simulink model "lab2_examples"  (R2022b)
settings: Solver=VariableStepAuto  StartTime=0.0  StopTime=10.0  RelTol=1e-3
settings Model: Creator=gaura  LastModifiedBy=gaura

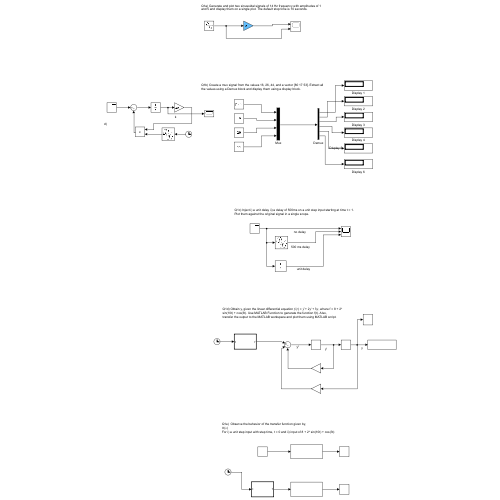
[thumbnail: Simulink's stored preview of the top-level diagram]
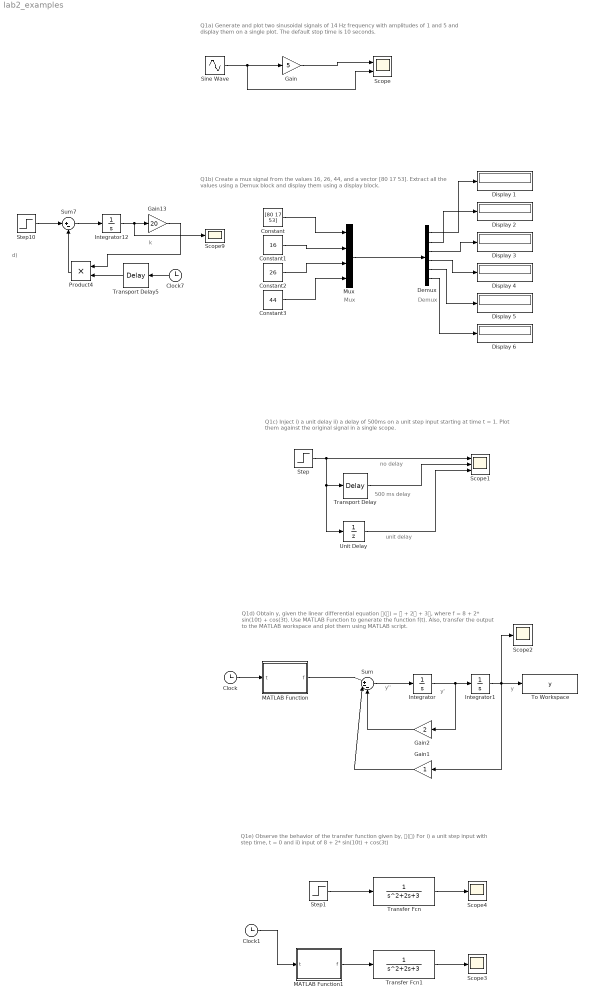
== system lab2_examples ==
  note: d)
  note: y''
  note: y
  note: Q1c) Inject i) a unit delay ii) a delay of 500ms on a unit step input starting at time t = 1. Plot them against the original signal in a single scope.
  note: Q1b) Create a mux signal from the values 16, 26, 44, and a vector [80 17 53]. Extract all the values using a Demux block and display them using a display block.
  note: k
  note: unit delay
  note: Demux
  note: 500 ms delay
  note: Mux
  note: Q1d) Obtain y, given the linear differential equation 𝑓(𝑡) = 𝑦̈ + 2𝑦̇ + 3𝑦, where f = 8 + 2* sin(10t) + cos(3t). Use MATLAB Function to generate the function f(t). Also,
      | transfer the output to the MATLAB workspace and plot them using MATLAB script.
  note: Q1e)  Observe the behavior of the transfer function given by,
      | 𝐻(𝑠)
      | For i) a unit step input with step time, t = 0 and ii) input of 8 + 2* sin(10t) + cos(3t)
  note: y'
  note: Q1a) Generate and plot two sinusoidal signals of 14 Hz frequency with amplitudes of 1 and 5 and display them on a single plot. The default stop time is 10 seconds.
  note: no delay
  Clock : Clock
  Clock1 : Clock
  Clock7 : Clock
  Constant : Constant  Value=[80 17 53]
  Constant1 : Constant  Value=16
  Constant2 : Constant  Value=26
  Constant3 : Constant  Value=44
  Demux : Demux  Outputs=6
  Display {1..6} (6 alike) : Display
  Gain : Gain  Gain=5
  Gain1 : Gain
  Gain13 : Gain  Gain=20
  Gain2 : Gain  Gain=2
  Integrator : Integrator
  Integrator1 : Integrator
  Integrator12 : Integrator
  MATLAB Function : MATLAB Function  TreatAsAtomicUnit=on
  MATLAB Function1 : MATLAB Function  TreatAsAtomicUnit=on
  Mux : Mux
  Product4 : Product
  Scope : Scope  NumInputPorts=2
  Scope1 : Scope  NumInputPorts=3
  Scope{2..4,9} (4 alike) : Scope
  Sine Wave : Sin  Frequency=14*2*pi  SampleTime=0
  Step : Step  SampleTime=0
  Step1 : Step  Time=0  SampleTime=0
  Step10 : Step  SampleTime=0
  Sum : Sum  Inputs=|+--
  Sum7 : Sum  Inputs=|+-
  To Workspace : ToWorkspace  VariableName=y  SaveFormat=Timeseries  SampleTime=-1
  Transfer Fcn : TransferFcn  Denominator=[1 2 3]
  Transfer Fcn1 : TransferFcn  Denominator=[1 2 3]
  Transport Delay : TransportDelay  DelayTime=0.5
  Transport Delay5 : TransportDelay  DelayTime=0.1
  Unit Delay : UnitDelay  SampleTime=0.25  HasFrameUpgradeWarning=on
  wires:
  Product4/1 -> Sum7/2
  Step10/1 -> Sum7/1
  Sum7/1 -> Integrator12/1
  Transport Delay5/1 -> Product4/2
  Gain/1 -> Scope/1
  Demux/5 -> Display 5/1
  Step1/1 -> Transfer Fcn/1
  MATLAB Function1/1(f) -> Transfer Fcn1/1
  Integrator1/1 -> Gain1/1, Scope2/1, To Workspace/1
  Demux/2 -> Display 2/1
  Clock/1 -> MATLAB Function/1(t)
  Gain13/1 -> Product4/1
  Transport Delay/1 -> Scope1/2
  Demux/3 -> Display 3/1
  Gain1/1 -> Sum/2
  Transfer Fcn1/1 -> Scope3/1
  Demux/6 -> Display 6/1
  Sum/1 -> Integrator/1
  Integrator/1 -> Gain2/1, Integrator1/1
  Demux/1 -> Display 1/1
  Integrator12/1 -> Scope9/1, Gain13/1
  Demux/4 -> Display 4/1
  Unit Delay/1 -> Scope1/3
  Gain2/1 -> Sum/3
  MATLAB Function/1(f) -> Sum/1
  Constant3/1 -> Mux/4
  Constant2/1 -> Mux/3
  Step/1 -> Unit Delay/1, Transport Delay/1, Scope1/1
  Mux/1 -> Demux/1
  Clock1/1 -> MATLAB Function1/1(t)
  Clock7/1 -> Transport Delay5/1
  Sine Wave/1 -> Scope/2, Gain/1
  Constant/1 -> Mux/1
  Transfer Fcn/1 -> Scope4/1
  Constant1/1 -> Mux/2

== matlab function lab2_examples/MATLAB Function ==
  data: t input; f output
function f = fcn(t)
    f = 8 + 2*sin(10*t)+cos(3*t);

== matlab function lab2_examples/MATLAB Function1 ==
  data: t input; f output
function f = fcn(t)
    f = 8 + 2*sin(10*t)+cos(3*t);
